simulink model "lateral_autopilot_3e"  (R2016b)
settings: Solver=VariableStepAuto  StartTime=0.0  StopTime=t_end  RelTol=1e-3
values from neighbouring files (symbols this model uses):
  A = [ -0.322 0.052 0.028 -1.12 0.002 ... (first row only)    [parameters_P3.m]
  B = [ 0 0 0 0 10]'    [parameters_P3.m]
  C = system_information_struct.C    [kalmann_filter.m]    (also in parameters_P3.m = [0 0 0 1 0)
  D = [0 0 0]'    [parameters_P3.m]
  d = 2*deg2rad    [run_task_3e.m]    (also in run_task_3f.m)
  delta_a_max = 25*deg2rad    (= 0.436332312999)    [parameters_P3.m]
  g = 9.81    [parameters_P3.m]
  h = 0.01    [parameters_P3.m]
  integrator_error_limit = 2*deg2rad    (= 0.0349065850399)    [parameters_P3.m]
  k_d_phi = (2*zeta_phi*omega_n_phi - a_phi_1) / a_phi_2    [parameters_P3.m]
  k_i_chi = omega_n_chi^2*V_g/g    [parameters_P3.m]
  k_i_phi = 0    [parameters_P3.m]
  k_p_chi = 2*zeta_chi*omega_n_chi*V_g/g    [parameters_P3.m]
  k_p_phi = sign(a_phi_2)*delta_a_max /e_phi_max    [parameters_P3.m]
  V_g = 637/3.6    (= 176.944444444)    [parameters_P3.m]
  var_p = (0.5*deg2rad)^2    (= 7.61543549467e-05)    [parameters_P3.m]
  var_phi = (0.2*deg2rad)^2    (= 1.21846967915e-05)    [parameters_P3.m]
  var_r = (2*deg2rad)^2    (= 0.00121846967915)    [parameters_P3.m]
settings Model: Creator=EllaLovise  LastModifiedBy=EllaLovise

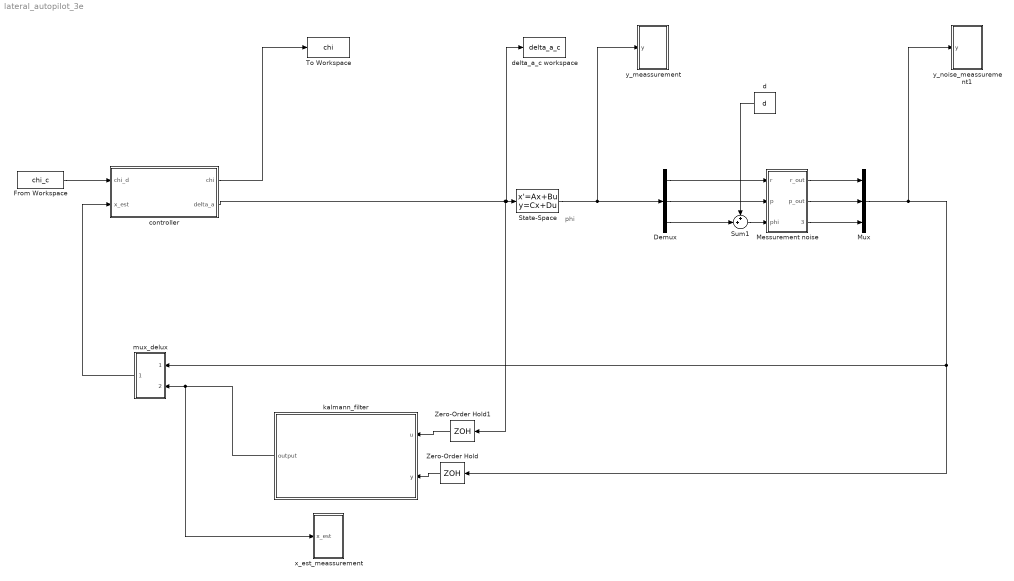
== system lateral_autopilot_3e ==
  note: phi
  Demux : Demux  Outputs=3
  From Workspace : FromWorkspace  VariableName=chi_c  OutputAfterFinalValue=Holding final value
  Messurement noise : Subsystem
  Mux : Mux  Inputs=3
  State-Space : StateSpace  A=A  B=B  C=C  D=D  X0=0
  Sum1 : Sum  Inputs=++|
  To Workspace : ToWorkspace  VariableName=chi  SaveFormat=Structure With Time  SampleTime=-1
  Zero-Order Hold : ZeroOrderHold  SampleTime=h
  Zero-Order Hold1 : ZeroOrderHold  SampleTime=h
  controller : Subsystem
  d : Constant  Value=d
  delta_a_c workspace : ToWorkspace  VariableName=delta_a_c  SaveFormat=Structure With Time  SampleTime=-1
  kalmann_filter : MATLAB Function  TreatAsAtomicUnit=on
  mux_delux : Subsystem
  x_est_meassurement : Subsystem
  y_meassurement : Subsystem
  y_noise_meassurement1 : Subsystem
  wires:
  State-Space/1 -> y_meassurement/1(y), Demux/1
  controller/1(chi) -> To Workspace/1
  From Workspace/1 -> controller/1(chi_d)
  Zero-Order Hold/1 -> kalmann_filter/2(y)
  Zero-Order Hold1/1 -> kalmann_filter/1(u)
  controller/2(delta_a) -> delta_a_c workspace/1, State-Space/1, Zero-Order Hold1/1
  Demux/1 -> Messurement noise/1(r)
  Demux/2 -> Messurement noise/2(p)
  Sum1/1 -> Messurement noise/3(phi)
  Messurement noise/1(r_out) -> Mux/1
  Messurement noise/2(p_out) -> Mux/2
  Messurement noise/3(phi_out) -> Mux/3
  d/1 -> Sum1/1
  Demux/3 -> Sum1/2
  Mux/1 -> y_noise_meassurement1/1(y), Zero-Order Hold/1, mux_delux/1(y_noise)
  kalmann_filter/1(output) -> x_est_meassurement/1(x_est), mux_delux/2(x_kalmann)
  mux_delux/1(x_est) -> controller/2(x_est)

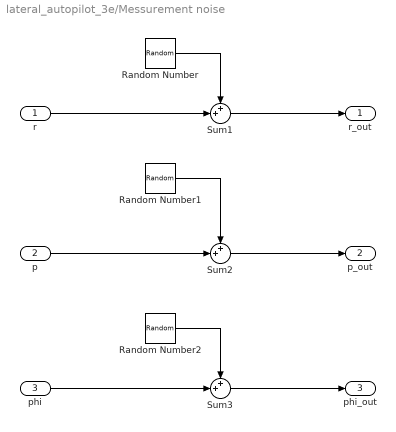
== system lateral_autopilot_3e/Messurement noise ==
  r : Inport
  p : Inport  Port=2
  phi : Inport  Port=3
  Random Number : RandomNumber  Variance=var_r
  Random Number1 : RandomNumber  Variance=var_p
  Random Number2 : RandomNumber  Variance=var_phi
  Sum1 : Sum  Inputs=++|
  Sum2 : Sum  Inputs=++|
  Sum3 : Sum  Inputs=++|
  r_out : Outport
  p_out : Outport  Port=2
  phi_out : Outport  Port=3
  wires:
  p/1 -> Sum2/2
  Sum1/1 -> r_out/1
  Sum2/1 -> p_out/1
  Sum3/1 -> phi_out/1
  Random Number/1 -> Sum1/1
  r/1 -> Sum1/2
  Random Number2/1 -> Sum3/1
  Random Number1/1 -> Sum2/1
  phi/1 -> Sum3/2

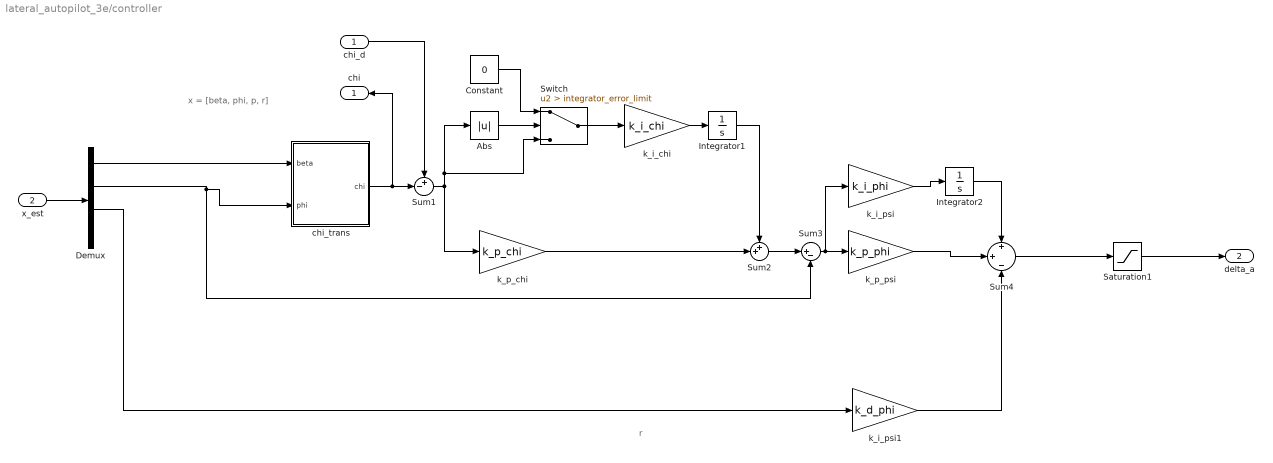
== system lateral_autopilot_3e/controller ==
  note: r
  note: x = [beta, phi, p, r]
  chi_d : Inport
  x_est : Inport  Port=2
  Abs : Abs
  Constant : Constant  Value=0
  Demux : Demux
  Integrator1 : Integrator
  Integrator2 : Integrator
  Saturation1 : Saturate  UpperLimit=delta_a_max  LowerLimit=-1*delta_a_max
  Sum1 : Sum  Inputs=+-|
  Sum2 : Sum  Inputs=++|
  Sum3 : Sum  Inputs=|+-
  Sum4 : Sum  Inputs=+|+|-
  Switch : Switch  Criteria=u2 > Threshold  Threshold=integrator_error_limit
  chi_trans : Subsystem
  k_i_chi : Gain  Gain=k_i_chi
  k_i_psi : Gain  Gain=k_i_phi
  k_i_psi1 : Gain  Gain=k_d_phi
  k_p_chi : Gain  Gain=k_p_chi
  k_p_psi : Gain  Gain=k_p_phi
  chi : Outport
  delta_a : Outport  Port=2
  wires:
  k_p_chi/1 -> Sum2/2
  Sum2/1 -> Sum3/1
  Sum3/1 -> k_p_psi/1, k_i_psi/1
  Integrator2/1 -> Sum4/1
  k_i_psi1/1 -> Sum4/3
  k_p_psi/1 -> Sum4/2
  k_i_psi/1 -> Integrator2/1
  Demux/3 -> k_i_psi1/1
  k_i_chi/1 -> Integrator1/1
  Integrator1/1 -> Sum2/1
  x_est/1 -> Demux/1
  Sum1/1 -> Abs/1, Switch/3, k_p_chi/1
  chi_trans/1(chi) -> chi/1, Sum1/2
  chi_d/1 -> Sum1/1
  Saturation1/1 -> delta_a/1
  Abs/1 -> Switch/2
  Switch/1 -> k_i_chi/1
  Constant/1 -> Switch/1
  Sum4/1 -> Saturation1/1
  Demux/2 -> chi_trans/2(phi), Sum3/2
  Demux/1 -> chi_trans/1(beta)

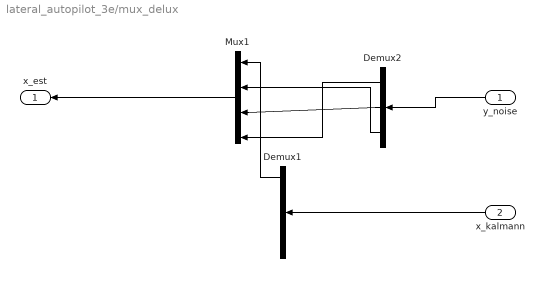
== system lateral_autopilot_3e/mux_delux ==
  y_noise : Inport
  x_kalmann : Inport  Port=2
  Demux1 : Demux
  Demux2 : Demux  Outputs=3
  Mux1 : Mux
  x_est : Outport
  wires:
  Demux2/2 -> Mux1/3
  x_kalmann/1 -> Demux1/1
  Demux2/3 -> Mux1/2
  y_noise/1 -> Demux2/1
  Mux1/1 -> x_est/1
  Demux2/1 -> Mux1/4
  Demux1/1 -> Mux1/1

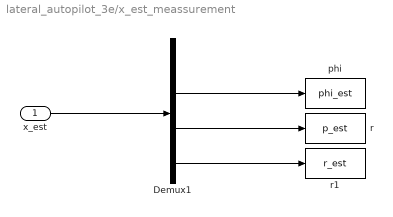
== system lateral_autopilot_3e/x_est_meassurement ==
  x_est : Inport
  Demux1 : Demux
  "phi " : ToWorkspace  VariableName=phi_est  SaveFormat=Structure With Time  SampleTime=-1
  r : ToWorkspace  VariableName=p_est  SaveFormat=Structure With Time  SampleTime=-1
  r1 : ToWorkspace  VariableName=r_est  SaveFormat=Structure With Time  SampleTime=-1
  wires:
  x_est/1 -> Demux1/1
  Demux1/2 -> "phi "/1
  Demux1/4 -> r1/1
  Demux1/3 -> r/1

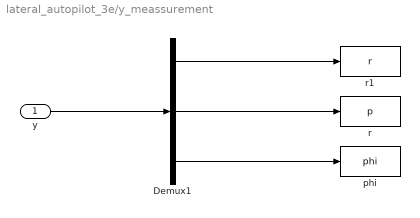
== system lateral_autopilot_3e/y_meassurement ==
  y : Inport
  Demux1 : Demux  Outputs=3
  "phi " : ToWorkspace  VariableName=phi  SaveFormat=Structure With Time  SampleTime=-1
  r : ToWorkspace  VariableName=p  SaveFormat=Structure With Time  SampleTime=-1
  r1 : ToWorkspace  VariableName=r  SaveFormat=Structure With Time  SampleTime=-1
  wires:
  y/1 -> Demux1/1
  Demux1/1 -> r1/1
  Demux1/2 -> r/1
  Demux1/3 -> "phi "/1

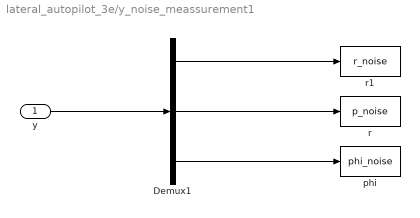
== system lateral_autopilot_3e/y_noise_meassurement1 ==
  y : Inport
  Demux1 : Demux  Outputs=3
  "phi " : ToWorkspace  VariableName=phi_noise  SaveFormat=Structure With Time  SampleTime=-1
  r : ToWorkspace  VariableName=p_noise  SaveFormat=Structure With Time  SampleTime=-1
  r1 : ToWorkspace  VariableName=r_noise  SaveFormat=Structure With Time  SampleTime=-1
  wires:
  y/1 -> Demux1/1
  Demux1/1 -> r1/1
  Demux1/2 -> r/1
  Demux1/3 -> "phi "/1

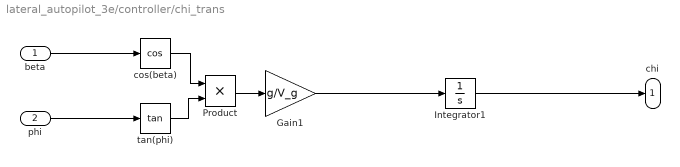
== system lateral_autopilot_3e/controller/chi_trans ==
  beta : Inport
  phi : Inport  Port=2
  Gain1 : Gain  Gain=g/V_g
  Integrator1 : Integrator
  Product : Product
  cos(beta) : Trigonometry  Operator=cos
  tan(phi) : Trigonometry  Operator=tan
  chi : Outport
  wires:
  phi/1 -> tan(phi)/1
  Integrator1/1 -> chi/1
  beta/1 -> cos(beta)/1
  tan(phi)/1 -> Product/2
  Product/1 -> Gain1/1
  cos(beta)/1 -> Product/1
  Gain1/1 -> Integrator1/1

== matlab function lateral_autopilot_3e/kalmann_filter ==
  data: u input; y input; output output; system_information_struct parameter
function output = fcn(u,y, system_information_struct)
persistent P_priori init_flag x_priori

A_d = system_information_struct.A_d;
B_d = system_information_struct.B_d;
E_d = system_information_struct.E_d;
C_d = system_information_struct.C_d;
Q = system_information_struct.Q;
I = system_information_struct.I;
R = system_information_struct.R;

if isempty(init_flag) %check if first round 
    init_flag = 1;
    
    P_0_priori= eye(4); 
    x_0_priori = [0; 0; 0; 0];
    P_priori = P_0_priori;
    x_priori = x_0_priori;
end

% 1) Compute Kalman gain
L = P_priori * C_d' * inv( C_d * P_priori * C_d' + R); 

% 2) update error covariance matrix
P = ( I - L*C_d)*P_priori*( I- L*C_d)' + L* R*L';

% 3) Update estimate with measurement
x_posteriori = x_priori + L * ( y - C_d*x_priori);

% 4) Project ahead
x_next_priori = A_d * x_posteriori + B_d*u;
P_next_priori = A_d*P*A_d' + E_d*Q*E_d';

x_priori = x_next_priori;
P_priori = P_next_priori; 

output = x_posteriori;
